simulink library "CTRL_SPECCTRL_FF_STEER"  (R2024b)
settings: Solver=VariableStepAuto  StartTime=0.0  StopTime=10.0  RelTol=1e-3
settings Model: Creator=blatak  LastModifiedBy=blatak

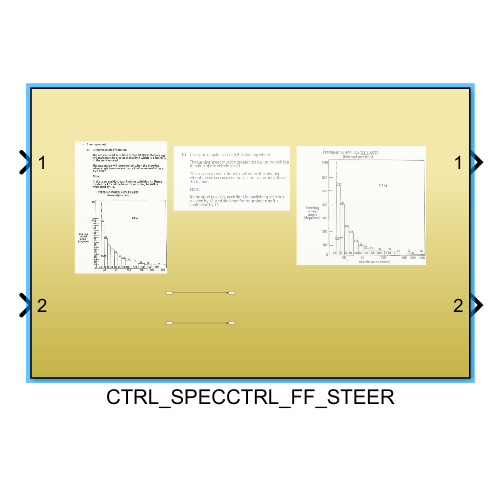
[thumbnail: Simulink's stored preview of the top-level diagram]
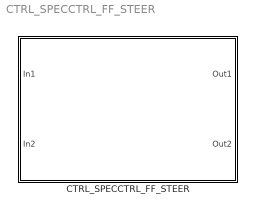
== system CTRL_SPECCTRL_FF_STEER ==
  CTRL_SPECCTRL_FF_STEER : Subsystem

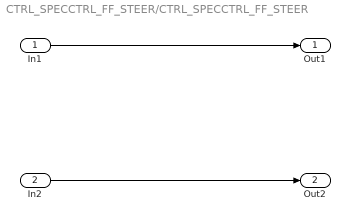
== system CTRL_SPECCTRL_FF_STEER/CTRL_SPECCTRL_FF_STEER ==
  In1 : Inport
  In2 : Inport  Port=2
  Out1 : Outport
  Out2 : Outport  Port=2
  wires:
  In2/1 -> Out2/1
  In1/1 -> Out1/1
